simulink model "food_bowl"  (R2023a)
settings: Solver=VariableStepAuto  StartTime=0.0  StopTime=100  RelTol=1e-4
model workspace (MAT data in the model file):
  K = 1
  a = Simulink.Parameter
  a.DataType = 'auto'
  a.Complexity = 'real'
  a.Dimensions = [0 0]
libraries: embmathops x1
settings Model: Creator=laurabryant  LastModifiedBy=laurabryant
settings DebuggingCC: AlgebraicLoopMsg=none

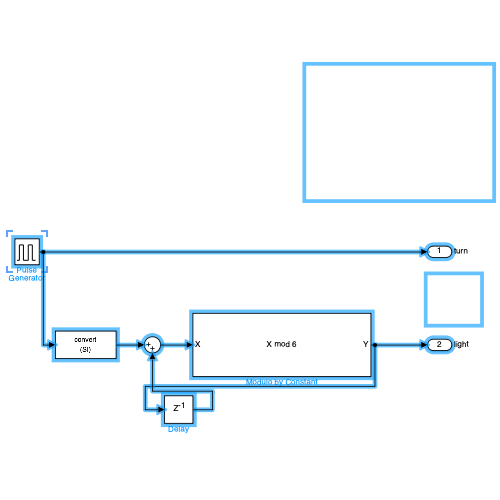
[thumbnail: Simulink's stored preview of the top-level diagram]
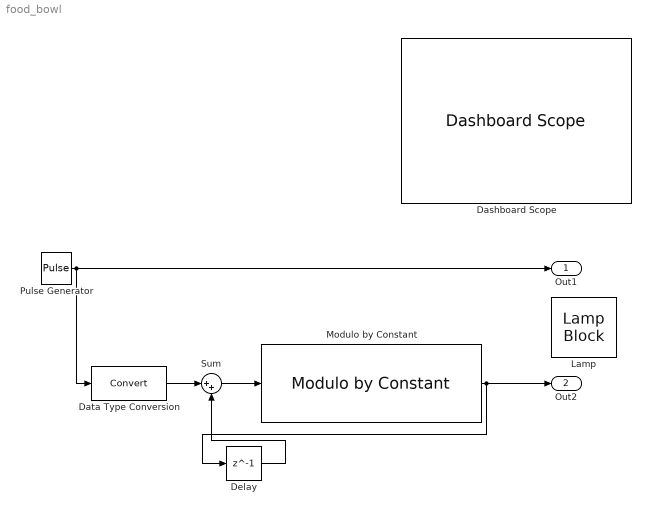
== system food_bowl ==
  Dashboard Scope : DashboardScope
  Data Type Conversion : DataTypeConversion  OutMin=0  OutMax=1  ConvertRealWorld=Stored Integer (SI)  RndMeth=Nearest  SaturateOnIntegerOverflow=off
  Delay : Delay  DelayLength=1  InitialCondition=0
  Lamp : LampBlock  LabelPosition=Hide
  Modulo by Constant : embmathops/Modulo by Constant  Denominator=6  SimulateUsing=Code generation
      settings: LibrarySourceBlock=embeddedMathLib/Modulo by Constant
  Pulse Generator : DiscretePulseGenerator  PulseType=Time based  Period=8  PulseWidth=2
  Sum : Sum  Inputs=|++
  Out1 : Outport  SignalName=turn
  Out2 : Outport  Port=2  SignalName=light
  wires:
  Pulse Generator/1 -> Data Type Conversion/1, Out1/1
  Modulo by Constant/1 -> Delay/1, Out2/1
  Data Type Conversion/1 -> Sum/1
  Sum/1 -> Modulo by Constant/1
  Delay/1 -> Sum/2
